simulink model "controller"  (R2024b)
settings: Solver=FixedStepAuto  StartTime=0.0  StopTime=10.0  FixedStep=1/100  RelTol=1e-3
settings Model: Creator=DAUIN-Win10  LastModifiedBy=WxxGr
settings OptimizationCC: ReuseModelBlockBuffer=off
settings DebuggingCC: UnconnectedInputMsg=warning  UnconnectedOutputMsg=warning  UnconnectedLineMsg=warning
settings ModelReferenceCC: EnableRefExpFcnMdlSchedulingChecks=on
settings RTWCC: GPUComputeCapability=3.5  DLArmComputeVersion=19.05

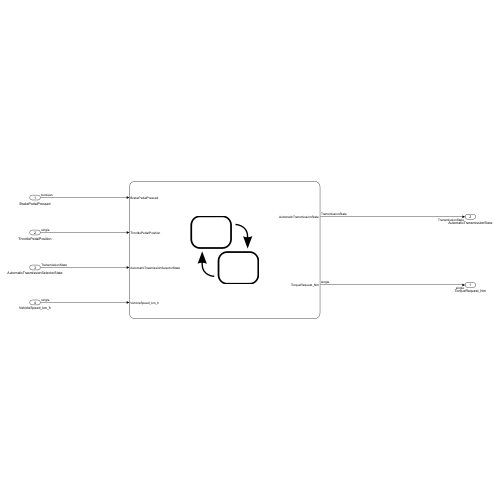
[thumbnail: Simulink's stored preview of the top-level diagram]
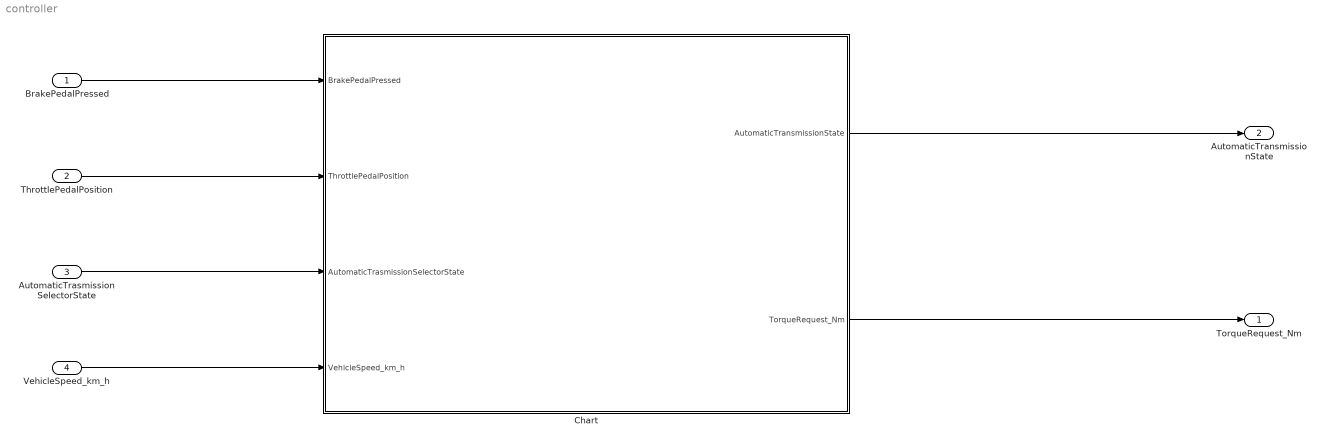
== system controller ==
  BrakePedalPressed : Inport  OutDataTypeStr=boolean
  ThrottlePedalPosition : Inport  Port=2  OutDataTypeStr=single
  AutomaticTrasmissionSelectorState : Inport  Port=3  OutDataTypeStr=Enum: TransmissionState
  VehicleSpeed_km_h : Inport  Port=4  OutDataTypeStr=single  Unit=km/h
  Chart : Stateflow chart  TreatAsAtomicUnit=on
  TorqueRequest_Nm : Outport  OutDataTypeStr=single  Unit=N*m
  AutomaticTransmissionState : Outport  Port=2  OutDataTypeStr=Enum: TransmissionState
  wires:
  BrakePedalPressed/1 -> Chart/1(BrakePedalPressed)
  ThrottlePedalPosition/1 -> Chart/2(ThrottlePedalPosition)
  AutomaticTrasmissionSelectorState/1 -> Chart/3(AutomaticTrasmissionSelectorState)
  VehicleSpeed_km_h/1 -> Chart/4(VehicleSpeed_km_h)
  Chart/1(AutomaticTransmissionState) -> AutomaticTransmissionState/1
  Chart/2(TorqueRequest_Nm) -> TorqueRequest_Nm/1

== stateflow chart controller/Chart ==
  state Park
    en:
    AutomaticTransmissionState =TransmissionState.Park;
    du:
    TorqueRequest_Nm = 0;
  state Brake
    en:
    AutomaticTransmissionState =TransmissionState.Brake;
    state BrakeNormal
      state brakeAccle
        du:
        TorqueRequest_Nm = single(ThrottlePedalPosition-1/3)*1.5 * 960/12;
      state barkDecele
        du:
        TorqueRequest_Nm = -3*single(1/3-ThrottlePedalPosition) * 960/12;
      state brak0Velocity
        du:
        %Add a PI controller
        error = 0 - VehicleSpeed_km_h;
        sumError = sumError + error;
        TorqueRequest_Nm = error*30+sumError*2;
        ex:sumError = 0;
      (default) -> brakeAccle
      brakeAccle -> barkDecele : [ThrottlePedalPosition<=1/3]
      barkDecele -> brakeAccle [order 1] : [ThrottlePedalPosition>1/3]
      (junction 83) -> brakeAccle
      barkDecele -> brak0Velocity [order 2] : [VehicleSpeed_km_h <= 0.2]
      brak0Velocity -> (junction 83) : [ThrottlePedalPosition>1/3]
    state barkStop
      en:
      TorqueRequest_Nm = 0;
    barkStop -> BrakeNormal : [BrakePedalPressed ~=1]
    BrakeNormal -> barkStop : [BrakePedalPressed ==1]
    (default) -> barkStop
  state Drive
    en:
    AutomaticTransmissionState =TransmissionState.Drive;
    state normalDrive
      du:
      TorqueRequest_Nm = single(ThrottlePedalPosition) * 960/12;
    state driveStop
      du:
      TorqueRequest_Nm = 0;
    normalDrive -> driveStop : [BrakePedalPressed ==1]
    driveStop -> normalDrive : [BrakePedalPressed~=1]
    (default) -> driveStop
  state Neutral
    en:
    AutomaticTransmissionState =TransmissionState.Neutral;
    du:
    TorqueRequest_Nm = 0;
  state Reverse
    en:
    AutomaticTransmissionState =TransmissionState.Reverse;
    state normalReverse
      du:
      TorqueRequest_Nm = -8*single(ThrottlePedalPosition) * 60/12;
    state reverseStop
      du:
      TorqueRequest_Nm = 0;
    normalReverse -> reverseStop : [BrakePedalPressed==1]
    reverseStop -> normalReverse : [BrakePedalPressed~=1]
    (default) -> reverseStop
  (default) -> Park
  Park -> Neutral : [BrakePedalPressed == 1 &&...
      | AutomaticTrasmissionSelectorState ~= TransmissionState.Park ]
  Neutral -> Park [order 1] : [VehicleSpeed_km_h<5 &&...
      | VehicleSpeed_km_h>-5 &&...
      | BrakePedalPressed == 1 &&...
      | AutomaticTrasmissionSelectorState == TransmissionState.Park ]
  Drive -> Neutral [order 1] : [AutomaticTrasmissionSelectorState ==TransmissionState.Neutral]
  Brake -> Drive : [AutomaticTrasmissionSelectorState ==TransmissionState.Drive||...
      | AutomaticTrasmissionSelectorState ==TransmissionState.Neutral]
  Neutral -> Reverse [order 2] : [VehicleSpeed_km_h<5 &&...
      | BrakePedalPressed == 1 &&...
      | AutomaticTrasmissionSelectorState ==TransmissionState.Reverse]
  Neutral -> Drive [order 3] : [VehicleSpeed_km_h>-5 &&...
      | BrakePedalPressed == 1 &&...
      | (AutomaticTrasmissionSelectorState ==TransmissionState.Drive||...
      | AutomaticTrasmissionSelectorState ==TransmissionState.Brake) ]
  Reverse -> Neutral : [AutomaticTrasmissionSelectorState  ~= TransmissionState.Reverse]
  Drive -> Brake [order 2] : [ThrottlePedalPosition>1/3 &&...
      | AutomaticTrasmissionSelectorState ==TransmissionState.Brake]
  data: AutomaticTransmissionState output; BrakePedalPressed input; ThrottlePedalPosition input; AutomaticTrasmissionSelectorState input; VehicleSpeed_km_h input; TorqueRequest_Nm output single; sumError local single =0; error local
